simulink library "monroe_library"  (R2012b)
settings: Solver=ode45  StartTime=0.0  StopTime=10.0  RelTol=1e-3
values from neighbouring files (symbols this model uses):
  input_bit_width = ', num2str(input_bit_width))    [fft_direct_draw.m]
undefined symbols (not defined in the file or in its folder): gcbh, xlBlockLoadCallback
libraries: xbsIndex_r4 x1880, monroe_library x159, casper_library x13, xps_library x1
(part 25 of 43)

== system monroe_library/direct_coeff_gen/coeff_gen_stage_3_group_4 ==
  sync : Inport
  Concat : xbsIndex_r4/Concat  num_inputs=2  dbl_ovrd=off  block_type=concat
  Concat1 : xbsIndex_r4/Concat  num_inputs=2  dbl_ovrd=off  block_type=concat
  Concat2 : xbsIndex_r4/Concat  num_inputs=2  dbl_ovrd=off  block_type=concat
  Constant : xbsIndex_r4/Constant  arith_type=Boolean  const=0  n_bits=16  bin_pt=14  explicit_period=on  period=1  equ=P=C  opselect=C  inp2=PCIN>>17  opr=+  inp1=P  carry=CIN  dbl_ovrd=off  block_type=constant
  Constant1 : xbsIndex_r4/Constant  arith_type=Boolean  const=1  n_bits=16  bin_pt=14  explicit_period=off  period=1  equ=P=C  opselect=C  inp2=PCIN>>17  opr=+  inp1=P  carry=CIN  dbl_ovrd=off  block_type=constant
  Constant3 : xbsIndex_r4/Constant  arith_type=Signed (2's comp)  const=0  n_bits=18  bin_pt=17  explicit_period=on  period=1  equ=P=C  opselect=C  inp2=PCIN>>17  opr=+  inp1=P  carry=CIN  dbl_ovrd=off  block_type=constant
  Constant4 : xbsIndex_r4/Constant  arith_type=Boolean  const=0  n_bits=16  bin_pt=14  explicit_period=off  period=1  equ=P=C  opselect=C  inp2=PCIN>>17  opr=+  inp1=P  carry=CIN  dbl_ovrd=off  block_type=constant
  Constant5 : xbsIndex_r4/Constant  arith_type=Unsigned  const=2  n_bits=10  bin_pt=0  explicit_period=on  period=1  equ=P=C  opselect=C  inp2=PCIN>>17  opr=+  inp1=P  carry=CIN  dbl_ovrd=off  block_type=constant
  Counter : xbsIndex_r4/Counter  cnt_type=Free Running  cnt_to=Inf  operation=Up  start_count=0  cnt_by_val=1  arith_type=Unsigned  n_bits=10  bin_pt=0  load_pin=on  rst=off  en=off  explicit_period=on  period=1  dbl_ovrd=off  use_behavioral_HDL=off  implementation=Fabric  block_type=counter
  Delay : xbsIndex_r4/Delay  en=off  latency=0  dbl_ovrd=off  reg_retiming=off  block_type=delay
  Dual Port RAM4 : xbsIndex_r4/Dual Port RAM  depth=2048  initVector=[-0.707106781186548 -0.70656422914471 -0.70602126144934 -0.705477878419852 -0.704934080375905 -0.704389867637401 -0.703845240524485 -0.703300199357549 -0.702754744457225 -0.702208876144392 -0.701662594740169 -0.701115900565919 -0.700568793943248 -0.700021275194006 -0.699473344640284 -0.698925002604414 -0.698376249408973 -0.697827085376777 -0.697277510830887 -0.696727526094601 -0.696177131491463 -0.695626327345255 -0.695075113980001 -0.694523491719966 -0.693971460889654 -0.693419021813812 -0.692866174817425 -0.692312920225718 -0.691759258364158 -0.691205189558448 -0.690650714134535 -0.6900958324186 -0.689540544737067 -0.688984851416597 -0.68842875278409 -0.687872249166686 -0.687315340891759 -0.686758028286926 -0.686200311680039 -0.685642191399188 -0.6850836677727 -0.684524741129142 -0.683965411797316 -0.683405680106259 -0.682845546385248 -0.682285010963796 -0.68172407417165 -0.681162736338796 -0.680600997795453 -0.680038858872079 -0.679476319899365 -0.678913381208238 -0.678350043129861 -0.677786305995632 -0.677222170137181 -0.676657635886375 -0.676092703575316 -0.675527373536339 -0.674961646102012 -0.674395521605139 -0.673829000378756 -0.673262082756133 -0.672694769070773 -0.672127059656412 -0.671558954847019 -0.670990454976794 -0.670421560380173 -0.669852271391821 -0.669282588346636 -0.668712511579748 -0.668142041426519 -0.66757117822254 -0.666999922303638 -0.666428274005865 -0.66585623366551 -0.665283801619087 -0.664710978203345 -0.66413776375526 -0.66356415861204 -0.662990163111121 -0.662415777590172 -0.661841002387087 -0.661265837839992 -0.660690284287242 -0.66011434206742 -0.659538011519339 -0.658961292982038 -0.658384186794785 -0.657806693297079 -0.657228812828643 -0.656650545729429 -0.656071892339618 -0.655492852999616 -0.654913428050056 -0.654333617831801 -0.653753422685936 -0.653172842953777 -0.652591878976863 -0.65201053109696 -0.65142879965606 -0.650846684996381 -0.650264187460366 -0.649681307390683 -0.649098045130226 -0.648514401022113 -0.647930375409685 -0.647345968636512 -0.646761181046384 -0.646176012983317 -0.645590464791549 -0.645004536815544 -0.644418229399988 -0.643831542889791 -0.643244477630086 -0.642657033966227 -0.642069212243793 -0.641481012808583 -0.640892436006621 -0.640303482184152 -0.639714151687641 -0.639124444863776 -0.638534362059467 -0.637943903621844 -0.637353069898259 -0.636761861236284 -0.636170277983712 -0.635578320488556 -0.63498598909905 -0.634393284163645 -0.633800206031017 -0.633206755050057 -0.632612931569878 -0.632018735939809 -0.631424168509402 -0.630829229628424 -0.630233919646865 -0.629638238914927 -0.629042187783036 -0.628445766601833 -0.627848975722177 -0.627251815495144 -0.62665428627203 -0.626056388404344 -0.625458122243814 -0.624859488142386 -0.624260486452221 -0.623661117525695 -0.623061381715401 -0.62246127937415 -0.621860810854965 -0.621259976511088 -0.620658776695972 -0.620057211763289 -0.619455282066924 -0.618852987960976 -0.61825032979976 -0.617647307937804 -0.61704392272985 -0.616440174530854 -0.615836063695985 -0.615231590580627 -0.614626755540375 -0.614021558931038 -0.613416001108639 -0.61281008242941 -0.612203803249798 -0.611597163926462 -0.610990164816272 -0.61038280627631 -0.609775088663869 -0.609167012336453 -0.608558577651779 -0.607949784967774 -0.607340634642573 -0.606731127034525 -0.606121262502186 -0.605511041404326 -0.60490046409992 -0.604289530948156 -0.603678242308431 -0.603066598540348 -0.602454600003724 -0.60184224705858 -0.601229540065149 -0.600616479383869 -0.600003065375389 -0.599389298400565 -0.598775178820459 -0.598160706996342 -0.597545883289693 -0.596930708062197 -0.596315181675744 -0.595699304492433 -0.59508307687457 -0.594466499184664 -0.593849571785434 -0.5932322950398 -0.592614669310891 -0.591996694962041 -0.591378372356788 -0.590759701858874 -0.590140683832249 -0.589521318641064 -0.588901606649676 -0.588281548222645 -0.587661143724737 -0.587040393520918 -0.586419297976361 -0.585797857456439 -0.585176072326731 -0.584553942953015 ...(+34827 chars)]  distributed_mem=Block RAM  init_a=0  init_b=0  rst_a=off  rst_b=off  en_a=off  en_b=off  latency=2  write_mode_A=No Read On Write  write_mode_B=No Read On Write  dbl_ovrd=off  optimize=Area  use_rpm=on  block_type=dpram
  Reinterpret : xbsIndex_r4/Reinterpret  force_arith_type=on  arith_type=Unsigned  force_bin_pt=on  bin_pt=0  block_type=reinterpret
      settings: infoedit="Changes signal type without altering the binary representation.   You can changed the signal between signed and unsigned, and relocate the binary point.<br><br>Hardware notes: In hardware this block costs nothing.<br><br>Example:  Suppose the input is 6 bits wide, signed, with 2 fractional bits, and the output is forced to unsigned with 0 fractional bits.  Then an input of -2.0 (1110.00 in binary 2's complement) becomes an output of 56 (111000 in binary)."
  Reinterpret1 : xbsIndex_r4/Reinterpret  force_arith_type=on  arith_type=Unsigned  force_bin_pt=on  bin_pt=0  block_type=reinterpret
      settings: infoedit="Changes signal type without altering the binary representation.   You can changed the signal between signed and unsigned, and relocate the binary point.<br><br>Hardware notes: In hardware this block costs nothing.<br><br>Example:  Suppose the input is 6 bits wide, signed, with 2 fractional bits, and the output is forced to unsigned with 0 fractional bits.  Then an input of -2.0 (1110.00 in binary 2's complement) becomes an output of 56 (111000 in binary)."
  count_slice : xbsIndex_r4/Slice  nbits=10  boolean_output=off  mode=Upper Bit Location + Width  bit1=0  base1=MSB of Input  bit0=0  base0=MSB of Input  dbl_ovrd=off  block_type=slice
  coeff : Outport
  wires:
  count_slice/1 -> Concat1/2, Concat/2  "xlsub2_Counter_out1"
  Constant3/1 -> Dual Port RAM4/5, Dual Port RAM4/2  "xlsub2_Constant3_out1"
  Constant/1 -> Dual Port RAM4/6, Dual Port RAM4/3  "xlsub2_Constant_out1"
  Reinterpret1/1 -> Concat2/2  "xlsub2_Reinterpret1_out1"
  Dual Port RAM4/2 -> Reinterpret1/1  "xlsub2_Dual_Port_RAM4_out2"
  Reinterpret/1 -> Concat2/1  "xlsub2_Reinterpret_out1"
  Dual Port RAM4/1 -> Reinterpret/1  "xlsub2_Dual_Port_RAM4_out1"
  Concat1/1 -> Dual Port RAM4/4  "xlsub2_Concat1_out1"
  Concat/1 -> Dual Port RAM4/1  "xlsub2_Concat_out1"
  Delay/1 -> coeff/1
  Concat2/1 -> Delay/1  "xlsub2_Concat2_out1"
  Counter/1 -> count_slice/1
  Constant5/1 -> Counter/2  "xlsub2_Constant5_out1"
  sync/1 -> Counter/1
  Constant4/1 -> Concat1/1  "xlsub2_Constant4_out1"
  Constant1/1 -> Concat/1  "xlsub2_Constant1_out1"

== system monroe_library/fft_direct_stage/uncram_coeff ==
  in : Inport
  signal1 : xbsIndex_r4/Slice  nbits=36  boolean_output=off  mode=Upper Bit Location + Width  bit1=-0  base1=MSB of Input  bit0=-0  base0=MSB of Input  dbl_ovrd=off  block_type=slice
  signal2 : xbsIndex_r4/Slice  nbits=36  boolean_output=off  mode=Upper Bit Location + Width  bit1=-36  base1=MSB of Input  bit0=-36  base0=MSB of Input  dbl_ovrd=off  block_type=slice
  signal3 : xbsIndex_r4/Slice  nbits=36  boolean_output=off  mode=Upper Bit Location + Width  bit1=-72  base1=MSB of Input  bit0=-72  base0=MSB of Input  dbl_ovrd=off  block_type=slice
  signal4 : xbsIndex_r4/Slice  nbits=36  boolean_output=off  mode=Upper Bit Location + Width  bit1=-108  base1=MSB of Input  bit0=-108  base0=MSB of Input  dbl_ovrd=off  block_type=slice
  signal5 : xbsIndex_r4/Slice  nbits=36  boolean_output=off  mode=Upper Bit Location + Width  bit1=-144  base1=MSB of Input  bit0=-144  base0=MSB of Input  dbl_ovrd=off  block_type=slice
  signal6 : xbsIndex_r4/Slice  nbits=36  boolean_output=off  mode=Upper Bit Location + Width  bit1=-180  base1=MSB of Input  bit0=-180  base0=MSB of Input  dbl_ovrd=off  block_type=slice
  signal7 : xbsIndex_r4/Slice  nbits=36  boolean_output=off  mode=Upper Bit Location + Width  bit1=-216  base1=MSB of Input  bit0=-216  base0=MSB of Input  dbl_ovrd=off  block_type=slice
  signal8 : xbsIndex_r4/Slice  nbits=36  boolean_output=off  mode=Upper Bit Location + Width  bit1=-252  base1=MSB of Input  bit0=-252  base0=MSB of Input  dbl_ovrd=off  block_type=slice
  out0 : Outport
  out1 : Outport  Port=2
  out2 : Outport  Port=3
  out3 : Outport  Port=4
  out4 : Outport  Port=5
  out5 : Outport  Port=6
  out6 : Outport  Port=7
  out7 : Outport  Port=8
  wires:
  in/1 -> signal8/1, signal7/1, signal6/1, signal5/1, signal4/1, signal3/1, signal2/1, signal1/1
  signal8/1 -> out7/1
  signal7/1 -> out6/1
  signal6/1 -> out5/1
  signal5/1 -> out4/1
  signal4/1 -> out3/1
  signal3/1 -> out2/1
  signal2/1 -> out1/1
  signal1/1 -> out0/1
